simulink model "ASKDemodulator"  (R2024a)
settings: Solver=VariableStepAuto  StartTime=0.0  StopTime=10.0  RelTol=1e-3
settings Model: Creator=prath  LastModifiedBy=prath

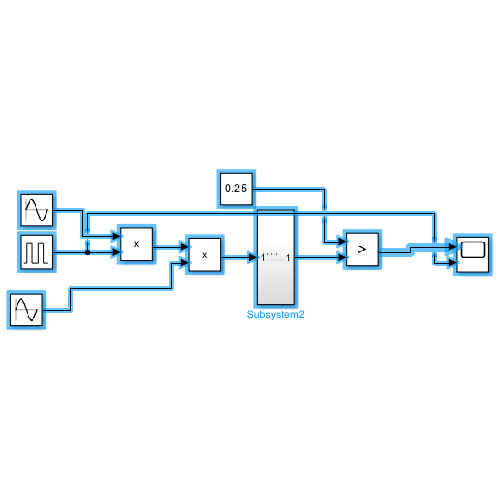
[thumbnail: Simulink's stored preview of the top-level diagram]
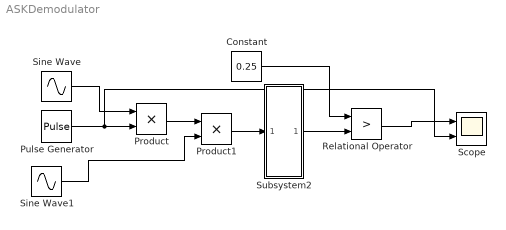
== system ASKDemodulator ==
  Constant : Constant  Value=0.25
  Product : Product
  Product1 : Product
  Pulse Generator : DiscretePulseGenerator  PulseType=Time based  Period=1  PulseWidth=50
  Relational Operator : RelationalOperator  Operator=>  OutDataTypeStr=boolean  RndMeth=Simplest  InputSameDT=off
  Scope : Scope  NumInputPorts=2
  Sine Wave : Sin  Frequency=100  SampleTime=0
  Sine Wave1 : Sin  Frequency=100  SampleTime=0
  Subsystem2 : Subsystem
  wires:
  Constant/1 -> Relational Operator/1
  Subsystem2/1(Out1) -> Relational Operator/2
  Sine Wave/1 -> Product/1
  Product1/1 -> Subsystem2/1(In1)
  Sine Wave1/1 -> Product1/2
  Product/1 -> Product1/1
  Pulse Generator/1 -> Scope/2, Product/2
  Relational Operator/1 -> Scope/1

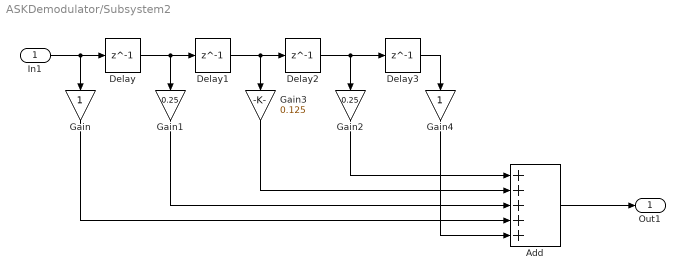
== system ASKDemodulator/Subsystem2 ==
  In1 : Inport
  Add : Sum  Inputs=+++++
  Delay{,1..3} (4 alike) : Delay  DelayLength=1
  Gain : Gain
  Gain1 : Gain  Gain=0.25
  Gain2 : Gain  Gain=0.25
  Gain3 : Gain  Gain=0.125
  Gain4 : Gain
  Out1 : Outport
  wires:
  Gain2/1 -> Add/1
  Gain1/1 -> Add/3
  Add/1 -> Out1/1
  Gain4/1 -> Add/5
  Delay/1 -> Delay1/1, Gain1/1
  Delay1/1 -> Delay2/1, Gain3/1
  In1/1 -> Gain/1, Delay/1
  Gain3/1 -> Add/2
  Delay2/1 -> Delay3/1, Gain2/1
  Delay3/1 -> Gain4/1
  Gain/1 -> Add/4
